simulink model "Shanthan_Heeirthan_EE469S3D_R45 (1)"  (R2023a)
settings: Solver=FixedStepDiscrete  StartTime=0.0  StopTime=120  FixedStep=dt0  RelTol=1e-3  EnableMultiTasking=on
PostLoadFcn:
  | %Set the size for the model
  | set_param(gcs,'Location',[10 10 1270 970])
  | %Set the zoom factor for the model
  | set_param(gcs,'ZoomFactor','100')
InitFcn:
  | tic
  | % Students Add call to their M-file HERE
  | Shanthan_Heeirthan_EE460_Final
  | INIT_S3D_01
StartFcn:
  | tend0=toc;
  | tic;
StopFcn:
  | tend=toc;
  | disp(['Simulation time = ' num2str(tout(end)) ' sec'])
  | disp(['Real time = ' num2str(tend) ' sec'])
  | title('DONE')
  | SCORE=round((max(0,120-tout(end)-tend0))*4+10*(40-FuelBurned)+sum(100*double(PDONE)-100*double(PDONE<.5)));
  | PlotS3D(PlotInput);
  | text(15,22,['S: ' num2str(SCORE)]);
values from neighbouring files (symbols this model uses):
  A = [0 1 0 0 0 0 ... (first row only)    [Shanthan_Heeirthan_EE460_Final (1).m]
  B = [0 0 0 ... (first row only)    [Shanthan_Heeirthan_EE460_Final (1).m]
  bm = [1 1 -1 -1 0 0 0 0; 0 0 0 0 -1 1 1 -1; -1 1 -1 1 3 -3 3 -3]    [Shanthan_Heeirthan_EE460_Final (1).m]
  C = [1 0 0 0 0 0 ... (first row only)    [Shanthan_Heeirthan_EE460_Final (1).m]
  D = [0 0 0 ... (first row only)    [Shanthan_Heeirthan_EE460_Final (1).m]
  Denchptheta = TFchptheta.Den{1}    [Shanthan_Heeirthan_EE460_Final (1).m]
  Denchpxy = TFchpxy.Den{1}    [Shanthan_Heeirthan_EE460_Final (1).m]
  Denclptheta = TFclptheta.Den{1}    [Shanthan_Heeirthan_EE460_Final (1).m]
  Denclpxy = TFclpxy.Den{1}    [Shanthan_Heeirthan_EE460_Final (1).m]
  Denlp = TFlp.Den{1}    [Shanthan_Heeirthan_EE460_Final (1).m]
  Kd = 2.1+0    (= 2.1)    [Shanthan_Heeirthan_EE460_Final (1).m]
  Ki = 0.0001    [Shanthan_Heeirthan_EE460_Final (1).m]
  Kp = 1.1+0.2    (= 1.3)    [Shanthan_Heeirthan_EE460_Final (1).m]
  L = place(A',C',ep)'    [Shanthan_Heeirthan_EE460_Final (1).m]
  Numchptheta = TFchptheta.Num{1}    [Shanthan_Heeirthan_EE460_Final (1).m]
  Numchpxy = TFchpxy.Num{1}    [Shanthan_Heeirthan_EE460_Final (1).m]
  Numclptheta = TFclptheta.Num{1}    [Shanthan_Heeirthan_EE460_Final (1).m]
  Numclpxy = TFclpxy.Num{1}    [Shanthan_Heeirthan_EE460_Final (1).m]
  Numlp = TFlp.Num{1}    [Shanthan_Heeirthan_EE460_Final (1).m]
  Pnewdata = [LVL.P1 LVL.P2 LVL.P3 LVL.P4]    [Shanthan_Heeirthan_EE460_Final (1).m]
  Sconfig = 1    [Shanthan_Heeirthan_EE460_Final (1).m]
  TFP1 = 2    [Shanthan_Heeirthan_EE460_Final (1).m]
  TFP1z = 1    [Shanthan_Heeirthan_EE460_Final (1).m]
  TFP2 = 2    [Shanthan_Heeirthan_EE460_Final (1).m]
  TFP2z = 1    [Shanthan_Heeirthan_EE460_Final (1).m]
  TFP3 = 2    [Shanthan_Heeirthan_EE460_Final (1).m]
  TFP3z = 1    [Shanthan_Heeirthan_EE460_Final (1).m]
  TFP4 = 2    [Shanthan_Heeirthan_EE460_Final (1).m]
  TFP4z = 1    [Shanthan_Heeirthan_EE460_Final (1).m]
  wcf = 2    [Shanthan_Heeirthan_EE460_Final (1).m]
  wcft = 10    [Shanthan_Heeirthan_EE460_Final (1).m]
undefined symbols (not defined in the file or in its folder): d2r, DiscIntNeverNeededParam, dt, dt0, fr, HM_S, HM_U, J, Jbase, JC0, L13, L24, LVL, M, M1, M2, M3, M4, mdti, Pdata, PTvec, r2d, SLIM, SQ, SSF, TOLdata, ULIM
libraries: simulink x85, aerolibanimutils x1, matrix_library x1
(part 4 of 7)

== system Shanthan_Heeirthan_EE469S3D_R45 (1)/S3D_Plant/Sensors/HealthMonitoring/Subsystem2 ==
  In1 : Inport
  Compare To Constant : simulink/Logic and Bit Operations/Compare To Constant  relop=>=  const=HM_S  OutDataTypeStr=boolean
  Constant : Constant  Value=0
  Constant1 : Constant
  Logical Operator : Logic  Operator=OR  AllPortsSameDT=off  OutDataTypeStr=boolean
  Sum : Sum  Inputs=|+-  OutDataTypeStr=int32
  Sum1 : Sum  Inputs=|++
  Switch : Switch  Criteria=u2 > Threshold  Threshold=eps  SaturateOnIntegerOverflow=off  InputSameDT=off
  Unit Delay : UnitDelay  SampleTime=dt0  HasFrameUpgradeWarning=on
  Unit Delay1 : UnitDelay  SampleTime=dt0  HasFrameUpgradeWarning=on
  Unit Delay2 : UnitDelay  SampleTime=dt0  HasFrameUpgradeWarning=on
  Out1 : Outport
  wires:
  Logical Operator/1 -> Unit Delay2/1, Out1/1
  Constant1/1 -> Sum1/1
  Compare To Constant/1 -> Logical Operator/1
  Switch/1 -> Unit Delay1/1, Compare To Constant/1
  In1/1 -> Sum/1, Unit Delay/1
  Unit Delay2/1 -> Logical Operator/2
  Unit Delay/1 -> Sum/2
  Sum/1 -> Switch/2
  Sum1/1 -> Switch/3
  Unit Delay1/1 -> Sum1/2
  Constant/1 -> Switch/1

== system Shanthan_Heeirthan_EE469S3D_R45 (1)/S3D_Plant/Sensors/HealthMonitoring/Subsystem3 ==
  In1 : Inport
  Compare To Constant : simulink/Logic and Bit Operations/Compare To Constant  relop=>=  const=HM_S  OutDataTypeStr=boolean
  Constant : Constant  Value=0
  Constant1 : Constant
  Logical Operator : Logic  Operator=OR  AllPortsSameDT=off  OutDataTypeStr=boolean
  Sum : Sum  Inputs=|+-  OutDataTypeStr=int32
  Sum1 : Sum  Inputs=|++
  Switch : Switch  Criteria=u2 > Threshold  Threshold=eps  SaturateOnIntegerOverflow=off  InputSameDT=off
  Unit Delay : UnitDelay  SampleTime=dt0  HasFrameUpgradeWarning=on
  Unit Delay1 : UnitDelay  SampleTime=dt0  HasFrameUpgradeWarning=on
  Unit Delay2 : UnitDelay  SampleTime=dt0  HasFrameUpgradeWarning=on
  Out1 : Outport
  wires:
  Constant/1 -> Switch/1
  Unit Delay1/1 -> Sum1/2
  Sum1/1 -> Switch/3
  Sum/1 -> Switch/2
  Unit Delay/1 -> Sum/2
  Unit Delay2/1 -> Logical Operator/2
  In1/1 -> Unit Delay/1, Sum/1
  Switch/1 -> Compare To Constant/1, Unit Delay1/1
  Compare To Constant/1 -> Logical Operator/1
  Constant1/1 -> Sum1/1
  Logical Operator/1 -> Out1/1, Unit Delay2/1

== system Shanthan_Heeirthan_EE469S3D_R45 (1)/S3D_Plant/Sensors/HealthMonitoring/Subsystem4 ==
  In1 : Inport
  Compare To Constant : simulink/Logic and Bit Operations/Compare To Constant  relop=>=  const=HM_S  OutDataTypeStr=boolean
  Constant : Constant  Value=0
  Constant1 : Constant
  Logical Operator : Logic  Operator=OR  AllPortsSameDT=off  OutDataTypeStr=boolean
  Sum : Sum  Inputs=|+-  OutDataTypeStr=int32
  Sum1 : Sum  Inputs=|++
  Switch : Switch  Criteria=u2 > Threshold  Threshold=eps  SaturateOnIntegerOverflow=off  InputSameDT=off
  Unit Delay : UnitDelay  SampleTime=dt0  HasFrameUpgradeWarning=on
  Unit Delay1 : UnitDelay  SampleTime=dt0  HasFrameUpgradeWarning=on
  Unit Delay2 : UnitDelay  SampleTime=dt0  HasFrameUpgradeWarning=on
  Out1 : Outport
  wires:
  Logical Operator/1 -> Unit Delay2/1, Out1/1
  Constant1/1 -> Sum1/1
  Compare To Constant/1 -> Logical Operator/1
  Switch/1 -> Unit Delay1/1, Compare To Constant/1
  In1/1 -> Sum/1, Unit Delay/1
  Unit Delay2/1 -> Logical Operator/2
  Unit Delay/1 -> Sum/2
  Sum/1 -> Switch/2
  Sum1/1 -> Switch/3
  Unit Delay1/1 -> Sum1/2
  Constant/1 -> Switch/1

== system Shanthan_Heeirthan_EE469S3D_R45 (1)/S3D_Plant/Sensors/HealthMonitoring/Subsystem5 ==
  In1 : Inport
  Compare To Constant : simulink/Logic and Bit Operations/Compare To Constant  relop=>=  const=HM_S  OutDataTypeStr=boolean
  Constant : Constant  Value=0
  Constant1 : Constant
  Logical Operator : Logic  Operator=OR  AllPortsSameDT=off  OutDataTypeStr=boolean
  Sum : Sum  Inputs=|+-  OutDataTypeStr=int32
  Sum1 : Sum  Inputs=|++
  Switch : Switch  Criteria=u2 > Threshold  Threshold=eps  SaturateOnIntegerOverflow=off  InputSameDT=off
  Unit Delay : UnitDelay  SampleTime=dt0  HasFrameUpgradeWarning=on
  Unit Delay1 : UnitDelay  SampleTime=dt0  HasFrameUpgradeWarning=on
  Unit Delay2 : UnitDelay  SampleTime=dt0  HasFrameUpgradeWarning=on
  Out1 : Outport
  wires:
  Constant/1 -> Switch/1
  Unit Delay1/1 -> Sum1/2
  Sum1/1 -> Switch/3
  Sum/1 -> Switch/2
  Unit Delay/1 -> Sum/2
  Unit Delay2/1 -> Logical Operator/2
  In1/1 -> Unit Delay/1, Sum/1
  Switch/1 -> Compare To Constant/1, Unit Delay1/1
  Compare To Constant/1 -> Logical Operator/1
  Constant1/1 -> Sum1/1
  Logical Operator/1 -> Out1/1, Unit Delay2/1

== system Shanthan_Heeirthan_EE469S3D_R45 (1)/S3D_Plant/Sensors/HealthMonitoring/Subsystem6 ==
  In1 : Inport
  Compare To Constant : simulink/Logic and Bit Operations/Compare To Constant  relop=>=  const=HM_S  OutDataTypeStr=boolean
  Constant : Constant  Value=0
  Constant1 : Constant
  Logical Operator : Logic  Operator=OR  AllPortsSameDT=off  OutDataTypeStr=boolean
  Sum : Sum  Inputs=|+-  OutDataTypeStr=int32
  Sum1 : Sum  Inputs=|++
  Switch : Switch  Criteria=u2 > Threshold  Threshold=eps  SaturateOnIntegerOverflow=off  InputSameDT=off
  Unit Delay : UnitDelay  SampleTime=dt0  HasFrameUpgradeWarning=on
  Unit Delay1 : UnitDelay  SampleTime=dt0  HasFrameUpgradeWarning=on
  Unit Delay2 : UnitDelay  SampleTime=dt0  HasFrameUpgradeWarning=on
  Out1 : Outport
  wires:
  Logical Operator/1 -> Unit Delay2/1, Out1/1
  Constant1/1 -> Sum1/1
  Compare To Constant/1 -> Logical Operator/1
  Switch/1 -> Unit Delay1/1, Compare To Constant/1
  In1/1 -> Sum/1, Unit Delay/1
  Unit Delay2/1 -> Logical Operator/2
  Unit Delay/1 -> Sum/2
  Sum/1 -> Switch/2
  Sum1/1 -> Switch/3
  Unit Delay1/1 -> Sum1/2
  Constant/1 -> Switch/1

== system Shanthan_Heeirthan_EE469S3D_R45 (1)/S3D_Plant/Sensors/HealthMonitoring/Subsystem7 ==
  In1 : Inport
  Compare To Constant : simulink/Logic and Bit Operations/Compare To Constant  relop=>=  const=HM_S  OutDataTypeStr=boolean
  Constant : Constant  Value=0
  Constant1 : Constant
  Logical Operator : Logic  Operator=OR  AllPortsSameDT=off  OutDataTypeStr=boolean
  Sum : Sum  Inputs=|+-  OutDataTypeStr=int32
  Sum1 : Sum  Inputs=|++
  Switch : Switch  Criteria=u2 > Threshold  Threshold=eps  SaturateOnIntegerOverflow=off  InputSameDT=off
  Unit Delay : UnitDelay  SampleTime=dt0  HasFrameUpgradeWarning=on
  Unit Delay1 : UnitDelay  SampleTime=dt0  HasFrameUpgradeWarning=on
  Unit Delay2 : UnitDelay  SampleTime=dt0  HasFrameUpgradeWarning=on
  Out1 : Outport
  wires:
  Constant/1 -> Switch/1
  Unit Delay1/1 -> Sum1/2
  Sum1/1 -> Switch/3
  Sum/1 -> Switch/2
  Unit Delay/1 -> Sum/2
  Unit Delay2/1 -> Logical Operator/2
  In1/1 -> Unit Delay/1, Sum/1
  Switch/1 -> Compare To Constant/1, Unit Delay1/1
  Compare To Constant/1 -> Logical Operator/1
  Constant1/1 -> Sum1/1
  Logical Operator/1 -> Out1/1, Unit Delay2/1

== system Shanthan_Heeirthan_EE469S3D_R45 (1)/S3D_Plant/Sensors/HealthMonitoring/Subsystem8 ==
  In1 : Inport
  Compare To Constant : simulink/Logic and Bit Operations/Compare To Constant  relop=>=  const=HM_S  OutDataTypeStr=boolean
  Constant : Constant  Value=0
  Constant1 : Constant
  Logical Operator : Logic  Operator=OR  AllPortsSameDT=off  OutDataTypeStr=boolean
  Sum : Sum  Inputs=|+-  OutDataTypeStr=int32
  Sum1 : Sum  Inputs=|++
  Switch : Switch  Criteria=u2 > Threshold  Threshold=eps  SaturateOnIntegerOverflow=off  InputSameDT=off
  Unit Delay : UnitDelay  SampleTime=dt0  HasFrameUpgradeWarning=on
  Unit Delay1 : UnitDelay  SampleTime=dt0  HasFrameUpgradeWarning=on
  Unit Delay2 : UnitDelay  SampleTime=dt0  HasFrameUpgradeWarning=on
  Out1 : Outport
  wires:
  Logical Operator/1 -> Unit Delay2/1, Out1/1
  Constant1/1 -> Sum1/1
  Compare To Constant/1 -> Logical Operator/1
  Switch/1 -> Unit Delay1/1, Compare To Constant/1
  In1/1 -> Sum/1, Unit Delay/1
  Unit Delay2/1 -> Logical Operator/2
  Unit Delay/1 -> Sum/2
  Sum/1 -> Switch/2
  Sum1/1 -> Switch/3
  Unit Delay1/1 -> Sum1/2
  Constant/1 -> Switch/1

== system Shanthan_Heeirthan_EE469S3D_R45 (1)/S3D_Plant/ThrusterValues/FailModes/Ufail1 ==
  Uin : Inport
  MP : Inport  Port=2
  Bus Selector1 : BusSelector  OutputSignals=U1cmd,U2cmd,U3cmd,U4cmd,U5cmd,U6cmd,U7cmd,U8cmd,U9cmd,U10cmd  OutputAsBus=on
  Bus Selector2 : BusSelector  OutputSignals=MfuelVector
  Bus to Vector2 : BusToVector
  CURRENT : Subsystem  TreatAsAtomicUnit=on
  Compare To Constant2 : simulink/Logic and Bit Operations/Compare To Constant  relop=>  const=eps  OutDataTypeStr=boolean
  Constant2 : Constant  Value=LVL.Uft(Udx,1)+rand*(LVL.Uft(Udx,2)-LVL.Uft(Udx,1))  SampleTime=dt0
  Constant3 : Constant  Value=LVL.Ufail(Udx)  SampleTime=dt0
  Constant4 : Constant  Value=-1  SampleTime=dt0
  Digital Clock : DigitalClock  SampleTime=dt0
  FailLogic : Subsystem
  If : If  IfExpression=u1 < -0.5  ElseIfExpressions=u1 > 0.5 & u1 < 1.5  SampleTime=dt0
  MAX : Subsystem  TreatAsAtomicUnit=on
  MIN : Subsystem  TreatAsAtomicUnit=on
  Merge : Merge  Inputs=3
  Relational Operator : RelationalOperator  Operator=<  OutDataTypeStr=boolean  InputSameDT=off
  Selector1 : Selector  InputPortWidth=4  IndexOptions=Index vector (dialog)  Indices=[Tank]  OutputSizes=1
  Selector2 : Selector  InputPortWidth=10  IndexOptions=Index vector (dialog)  Indices=[Udx]  OutputSizes=1
  Switch : Switch  Criteria=u2 > Threshold  SaturateOnIntegerOverflow=off  InputSameDT=off
  Switch1 : Switch  Criteria=u2 > Threshold  SaturateOnIntegerOverflow=off  InputSameDT=off
  Unit Delay : UnitDelay  SampleTime=dt0  HasFrameUpgradeWarning=on
  Uout : Outport
  wires:
  Selector2/1 -> Switch/1
  Bus to Vector2/1 -> Selector2/1
  FailLogic/1(NoFail) -> Switch/2
  Compare To Constant2/1 -> Switch1/2, FailLogic/2(FuelRemaining)
  Relational Operator/1 -> FailLogic/1(BeforeFail)
  Constant4/1 -> Switch1/3
  Constant3/1 -> Switch1/1
  Selector1/1 -> Compare To Constant2/1
  Bus Selector2/1 -> Selector1/1  "<MfuelVector>"
  MP/1 -> Bus Selector2/1
  Bus Selector1/1 -> Bus to Vector2/1
  Switch/1 -> Unit Delay/1, Uout/1
  Switch1/1 -> If/1, FailLogic/3(FailMode)
  Uin/1 -> Bus Selector1/1
  Merge/1 -> Switch/3
  MIN/1(Out1) -> Merge/1
  CURRENT/1(Out1) -> Merge/3
  Constant2/1 -> Relational Operator/2
  MAX/1(Out1) -> Merge/2
  Unit Delay/1 -> CURRENT/1(In1)
  If/3 -> CURRENT/Action
  Digital Clock/1 -> Relational Operator/1
  If/2 -> MAX/Action
  If/1 -> MIN/Action

== system Shanthan_Heeirthan_EE469S3D_R45 (1)/S3D_Plant/ThrusterValues/FailModes/Ufail10 ==
  Uin : Inport
  Bus Selector1 : BusSelector  OutputSignals=U1cmd,U2cmd,U3cmd,U4cmd,U5cmd,U6cmd,U7cmd,U8cmd,U9cmd,U10cmd  OutputAsBus=on
  Bus to Vector2 : BusToVector
  CURRENT : Subsystem  TreatAsAtomicUnit=on
  Constant1 : Constant  OutDataTypeStr=boolean  SampleTime=dt0
  Constant2 : Constant  Value=LVL.Uft(Udx,1)+rand*(LVL.Uft(Udx,2)-LVL.Uft(Udx,1))  SampleTime=dt0
  Constant3 : Constant  Value=LVL.Ufail(Udx)  SampleTime=dt0
  Constant4 : Constant  Value=-1  SampleTime=dt0
  Digital Clock : DigitalClock  SampleTime=dt0
  FailLogic : Subsystem
  If : If  IfExpression=u1 < -0.5  ElseIfExpressions=u1 > 0.5 & u1 < 1.5  SampleTime=dt0
  MAX : Subsystem  TreatAsAtomicUnit=on
  MIN : Subsystem  TreatAsAtomicUnit=on
  Merge : Merge  Inputs=3
  Relational Operator : RelationalOperator  Operator=<  OutDataTypeStr=boolean  InputSameDT=off
  Selector2 : Selector  InputPortWidth=10  IndexOptions=Index vector (dialog)  Indices=[Udx]  OutputSizes=1
  Switch : Switch  Criteria=u2 > Threshold  SaturateOnIntegerOverflow=off  InputSameDT=off
  Switch1 : Switch  Criteria=u2 > Threshold  SaturateOnIntegerOverflow=off  InputSameDT=off
  Unit Delay : UnitDelay  SampleTime=dt0  HasFrameUpgradeWarning=on
  Uout : Outport
  wires:
  Selector2/1 -> Switch/1
  Bus to Vector2/1 -> Selector2/1
  Bus Selector1/1 -> Bus to Vector2/1
  FailLogic/1(NoFail) -> Switch/2
  Constant1/1 -> Switch1/2, FailLogic/2(FuelRemaining)
  Relational Operator/1 -> FailLogic/1(BeforeFail)
  Constant4/1 -> Switch1/3
  Constant3/1 -> Switch1/1
  Switch/1 -> Unit Delay/1, Uout/1
  Switch1/1 -> If/1, FailLogic/3(FailMode)
  Uin/1 -> Bus Selector1/1
  Merge/1 -> Switch/3
  MIN/1(Out1) -> Merge/1
  CURRENT/1(Out1) -> Merge/3
  Constant2/1 -> Relational Operator/2
  MAX/1(Out1) -> Merge/2
  Unit Delay/1 -> CURRENT/1(In1)
  If/3 -> CURRENT/Action
  Digital Clock/1 -> Relational Operator/1
  If/2 -> MAX/Action
  If/1 -> MIN/Action

== system Shanthan_Heeirthan_EE469S3D_R45 (1)/S3D_Plant/ThrusterValues/FailModes/Ufail2 ==
  Uin : Inport
  MP : Inport  Port=2
  Bus Selector1 : BusSelector  OutputSignals=U1cmd,U2cmd,U3cmd,U4cmd,U5cmd,U6cmd,U7cmd,U8cmd,U9cmd,U10cmd  OutputAsBus=on
  Bus Selector2 : BusSelector  OutputSignals=MfuelVector
  Bus to Vector2 : BusToVector
  CURRENT : Subsystem  TreatAsAtomicUnit=on
  Compare To Constant2 : simulink/Logic and Bit Operations/Compare To Constant  relop=>  const=eps  OutDataTypeStr=boolean
  Constant2 : Constant  Value=LVL.Uft(Udx,1)+rand*(LVL.Uft(Udx,2)-LVL.Uft(Udx,1))  SampleTime=dt0
  Constant3 : Constant  Value=LVL.Ufail(Udx)  SampleTime=dt0
  Constant4 : Constant  Value=-1  SampleTime=dt0
  Digital Clock : DigitalClock  SampleTime=dt0
  FailLogic : Subsystem
  If : If  IfExpression=u1 < -0.5  ElseIfExpressions=u1 > 0.5 & u1 < 1.5  SampleTime=dt0
  MAX : Subsystem  TreatAsAtomicUnit=on
  MIN : Subsystem  TreatAsAtomicUnit=on
  Merge : Merge  Inputs=3
  Relational Operator : RelationalOperator  Operator=<  OutDataTypeStr=boolean  InputSameDT=off
  Selector1 : Selector  InputPortWidth=4  IndexOptions=Index vector (dialog)  Indices=[Tank]  OutputSizes=1
  Selector2 : Selector  InputPortWidth=10  IndexOptions=Index vector (dialog)  Indices=[Udx]  OutputSizes=1
  Switch : Switch  Criteria=u2 > Threshold  SaturateOnIntegerOverflow=off  InputSameDT=off
  Switch1 : Switch  Criteria=u2 > Threshold  SaturateOnIntegerOverflow=off  InputSameDT=off
  Unit Delay : UnitDelay  SampleTime=dt0  HasFrameUpgradeWarning=on
  Uout : Outport
  wires:
  Selector2/1 -> Switch/1
  Bus to Vector2/1 -> Selector2/1
  Bus Selector1/1 -> Bus to Vector2/1
  FailLogic/1(NoFail) -> Switch/2
  Compare To Constant2/1 -> Switch1/2, FailLogic/2(FuelRemaining)
  Relational Operator/1 -> FailLogic/1(BeforeFail)
  Constant4/1 -> Switch1/3
  Constant3/1 -> Switch1/1
  Selector1/1 -> Compare To Constant2/1
  Bus Selector2/1 -> Selector1/1  "<MfuelVector>"
  MP/1 -> Bus Selector2/1
  Switch/1 -> Unit Delay/1, Uout/1
  Switch1/1 -> If/1, FailLogic/3(FailMode)
  Uin/1 -> Bus Selector1/1
  Merge/1 -> Switch/3
  MIN/1(Out1) -> Merge/1
  CURRENT/1(Out1) -> Merge/3
  Constant2/1 -> Relational Operator/2
  MAX/1(Out1) -> Merge/2
  Unit Delay/1 -> CURRENT/1(In1)
  If/3 -> CURRENT/Action
  Digital Clock/1 -> Relational Operator/1
  If/2 -> MAX/Action
  If/1 -> MIN/Action

== system Shanthan_Heeirthan_EE469S3D_R45 (1)/S3D_Plant/ThrusterValues/FailModes/Ufail3 ==
  Uin : Inport
  MP : Inport  Port=2
  Bus Selector1 : BusSelector  OutputSignals=U1cmd,U2cmd,U3cmd,U4cmd,U5cmd,U6cmd,U7cmd,U8cmd,U9cmd,U10cmd  OutputAsBus=on
  Bus Selector2 : BusSelector  OutputSignals=MfuelVector
  Bus to Vector2 : BusToVector
  CURRENT : Subsystem  TreatAsAtomicUnit=on
  Compare To Constant2 : simulink/Logic and Bit Operations/Compare To Constant  relop=>  const=eps  OutDataTypeStr=boolean
  Constant2 : Constant  Value=LVL.Uft(Udx,1)+rand*(LVL.Uft(Udx,2)-LVL.Uft(Udx,1))  SampleTime=dt0
  Constant3 : Constant  Value=LVL.Ufail(Udx)  SampleTime=dt0
  Constant4 : Constant  Value=-1  SampleTime=dt0
  Digital Clock : DigitalClock  SampleTime=dt0
  FailLogic : Subsystem
  If : If  IfExpression=u1 < -0.5  ElseIfExpressions=u1 > 0.5 & u1 < 1.5  SampleTime=dt0
  MAX : Subsystem  TreatAsAtomicUnit=on
  MIN : Subsystem  TreatAsAtomicUnit=on
  Merge : Merge  Inputs=3
  Relational Operator : RelationalOperator  Operator=<  OutDataTypeStr=boolean  InputSameDT=off
  Selector1 : Selector  InputPortWidth=4  IndexOptions=Index vector (dialog)  Indices=[Tank]  OutputSizes=1
  Selector2 : Selector  InputPortWidth=10  IndexOptions=Index vector (dialog)  Indices=[Udx]  OutputSizes=1
  Switch : Switch  Criteria=u2 > Threshold  SaturateOnIntegerOverflow=off  InputSameDT=off
  Switch1 : Switch  Criteria=u2 > Threshold  SaturateOnIntegerOverflow=off  InputSameDT=off
  Unit Delay : UnitDelay  SampleTime=dt0  HasFrameUpgradeWarning=on
  Uout : Outport
  wires:
  Selector2/1 -> Switch/1
  Bus to Vector2/1 -> Selector2/1
  Bus Selector1/1 -> Bus to Vector2/1
  FailLogic/1(NoFail) -> Switch/2
  Compare To Constant2/1 -> Switch1/2, FailLogic/2(FuelRemaining)
  Relational Operator/1 -> FailLogic/1(BeforeFail)
  Constant4/1 -> Switch1/3
  Constant3/1 -> Switch1/1
  Selector1/1 -> Compare To Constant2/1
  Bus Selector2/1 -> Selector1/1  "<MfuelVector>"
  MP/1 -> Bus Selector2/1
  Switch/1 -> Unit Delay/1, Uout/1
  Switch1/1 -> If/1, FailLogic/3(FailMode)
  Uin/1 -> Bus Selector1/1
  Merge/1 -> Switch/3
  MIN/1(Out1) -> Merge/1
  CURRENT/1(Out1) -> Merge/3
  Constant2/1 -> Relational Operator/2
  MAX/1(Out1) -> Merge/2
  Unit Delay/1 -> CURRENT/1(In1)
  If/3 -> CURRENT/Action
  Digital Clock/1 -> Relational Operator/1
  If/2 -> MAX/Action
  If/1 -> MIN/Action

== system Shanthan_Heeirthan_EE469S3D_R45 (1)/S3D_Plant/ThrusterValues/FailModes/Ufail4 ==
  Uin : Inport
  MP : Inport  Port=2
  Bus Selector1 : BusSelector  OutputSignals=U1cmd,U2cmd,U3cmd,U4cmd,U5cmd,U6cmd,U7cmd,U8cmd,U9cmd,U10cmd  OutputAsBus=on
  Bus Selector2 : BusSelector  OutputSignals=MfuelVector
  Bus to Vector2 : BusToVector
  CURRENT : Subsystem  TreatAsAtomicUnit=on
  Compare To Constant2 : simulink/Logic and Bit Operations/Compare To Constant  relop=>  const=eps  OutDataTypeStr=boolean
  Constant2 : Constant  Value=LVL.Uft(Udx,1)+rand*(LVL.Uft(Udx,2)-LVL.Uft(Udx,1))  SampleTime=dt0
  Constant3 : Constant  Value=LVL.Ufail(Udx)  SampleTime=dt0
  Constant4 : Constant  Value=-1  SampleTime=dt0
  Digital Clock : DigitalClock  SampleTime=dt0
  FailLogic : Subsystem
  If : If  IfExpression=u1 < -0.5  ElseIfExpressions=u1 > 0.5 & u1 < 1.5  SampleTime=dt0
  MAX : Subsystem  TreatAsAtomicUnit=on
  MIN : Subsystem  TreatAsAtomicUnit=on
  Merge : Merge  Inputs=3
  Relational Operator : RelationalOperator  Operator=<  OutDataTypeStr=boolean  InputSameDT=off
  Selector1 : Selector  InputPortWidth=4  IndexOptions=Index vector (dialog)  Indices=[Tank]  OutputSizes=1
  Selector2 : Selector  InputPortWidth=10  IndexOptions=Index vector (dialog)  Indices=[Udx]  OutputSizes=1
  Switch : Switch  Criteria=u2 > Threshold  SaturateOnIntegerOverflow=off  InputSameDT=off
  Switch1 : Switch  Criteria=u2 > Threshold  SaturateOnIntegerOverflow=off  InputSameDT=off
  Unit Delay : UnitDelay  SampleTime=dt0  HasFrameUpgradeWarning=on
  Uout : Outport
  wires:
  Selector2/1 -> Switch/1
  Bus to Vector2/1 -> Selector2/1
  Bus Selector1/1 -> Bus to Vector2/1
  FailLogic/1(NoFail) -> Switch/2
  Compare To Constant2/1 -> Switch1/2, FailLogic/2(FuelRemaining)
  Relational Operator/1 -> FailLogic/1(BeforeFail)
  Constant4/1 -> Switch1/3
  Constant3/1 -> Switch1/1
  Selector1/1 -> Compare To Constant2/1
  Bus Selector2/1 -> Selector1/1  "<MfuelVector>"
  MP/1 -> Bus Selector2/1
  Switch/1 -> Unit Delay/1, Uout/1
  Switch1/1 -> If/1, FailLogic/3(FailMode)
  Uin/1 -> Bus Selector1/1
  Merge/1 -> Switch/3
  MIN/1(Out1) -> Merge/1
  CURRENT/1(Out1) -> Merge/3
  Constant2/1 -> Relational Operator/2
  MAX/1(Out1) -> Merge/2
  Unit Delay/1 -> CURRENT/1(In1)
  If/3 -> CURRENT/Action
  Digital Clock/1 -> Relational Operator/1
  If/2 -> MAX/Action
  If/1 -> MIN/Action

== system Shanthan_Heeirthan_EE469S3D_R45 (1)/S3D_Plant/ThrusterValues/FailModes/Ufail5 ==
  Uin : Inport
  MP : Inport  Port=2
  Bus Selector1 : BusSelector  OutputSignals=U1cmd,U2cmd,U3cmd,U4cmd,U5cmd,U6cmd,U7cmd,U8cmd,U9cmd,U10cmd  OutputAsBus=on
  Bus Selector2 : BusSelector  OutputSignals=MfuelVector
  Bus to Vector2 : BusToVector
  CURRENT : Subsystem  TreatAsAtomicUnit=on
  Compare To Constant2 : simulink/Logic and Bit Operations/Compare To Constant  relop=>  const=eps  OutDataTypeStr=boolean
  Constant2 : Constant  Value=LVL.Uft(Udx,1)+rand*(LVL.Uft(Udx,2)-LVL.Uft(Udx,1))  SampleTime=dt0
  Constant3 : Constant  Value=LVL.Ufail(Udx)  SampleTime=dt0
  Constant4 : Constant  Value=-1  SampleTime=dt0
  Digital Clock : DigitalClock  SampleTime=dt0
  FailLogic : Subsystem
  If : If  IfExpression=u1 < -0.5  ElseIfExpressions=u1 > 0.5 & u1 < 1.5  SampleTime=dt0
  MAX : Subsystem  TreatAsAtomicUnit=on
  MIN : Subsystem  TreatAsAtomicUnit=on
  Merge : Merge  Inputs=3
  Relational Operator : RelationalOperator  Operator=<  OutDataTypeStr=boolean  InputSameDT=off
  Selector1 : Selector  InputPortWidth=4  IndexOptions=Index vector (dialog)  Indices=[Tank]  OutputSizes=1
  Selector2 : Selector  InputPortWidth=10  IndexOptions=Index vector (dialog)  Indices=[Udx]  OutputSizes=1
  Switch : Switch  Criteria=u2 > Threshold  SaturateOnIntegerOverflow=off  InputSameDT=off
  Switch1 : Switch  Criteria=u2 > Threshold  SaturateOnIntegerOverflow=off  InputSameDT=off
  Unit Delay : UnitDelay  SampleTime=dt0  HasFrameUpgradeWarning=on
  Uout : Outport
  wires:
  Selector2/1 -> Switch/1
  Bus to Vector2/1 -> Selector2/1
  Bus Selector1/1 -> Bus to Vector2/1
  FailLogic/1(NoFail) -> Switch/2
  Compare To Constant2/1 -> Switch1/2, FailLogic/2(FuelRemaining)
  Relational Operator/1 -> FailLogic/1(BeforeFail)
  Constant4/1 -> Switch1/3
  Constant3/1 -> Switch1/1
  Selector1/1 -> Compare To Constant2/1
  Bus Selector2/1 -> Selector1/1  "<MfuelVector>"
  MP/1 -> Bus Selector2/1
  Switch/1 -> Unit Delay/1, Uout/1
  Switch1/1 -> If/1, FailLogic/3(FailMode)
  Uin/1 -> Bus Selector1/1
  Merge/1 -> Switch/3
  MIN/1(Out1) -> Merge/1
  CURRENT/1(Out1) -> Merge/3
  Constant2/1 -> Relational Operator/2
  MAX/1(Out1) -> Merge/2
  Unit Delay/1 -> CURRENT/1(In1)
  If/3 -> CURRENT/Action
  Digital Clock/1 -> Relational Operator/1
  If/2 -> MAX/Action
  If/1 -> MIN/Action

== system Shanthan_Heeirthan_EE469S3D_R45 (1)/S3D_Plant/ThrusterValues/FailModes/Ufail6 ==
  Uin : Inport
  MP : Inport  Port=2
  Bus Selector1 : BusSelector  OutputSignals=U1cmd,U2cmd,U3cmd,U4cmd,U5cmd,U6cmd,U7cmd,U8cmd,U9cmd,U10cmd  OutputAsBus=on
  Bus Selector2 : BusSelector  OutputSignals=MfuelVector
  Bus to Vector2 : BusToVector
  CURRENT : Subsystem  TreatAsAtomicUnit=on
  Compare To Constant2 : simulink/Logic and Bit Operations/Compare To Constant  relop=>  const=eps  OutDataTypeStr=boolean
  Constant2 : Constant  Value=LVL.Uft(Udx,1)+rand*(LVL.Uft(Udx,2)-LVL.Uft(Udx,1))  SampleTime=dt0
  Constant3 : Constant  Value=LVL.Ufail(Udx)  SampleTime=dt0
  Constant4 : Constant  Value=-1  SampleTime=dt0
  Digital Clock : DigitalClock  SampleTime=dt0
  FailLogic : Subsystem
  If : If  IfExpression=u1 < -0.5  ElseIfExpressions=u1 > 0.5 & u1 < 1.5  SampleTime=dt0
  MAX : Subsystem  TreatAsAtomicUnit=on
  MIN : Subsystem  TreatAsAtomicUnit=on
  Merge : Merge  Inputs=3
  Relational Operator : RelationalOperator  Operator=<  OutDataTypeStr=boolean  InputSameDT=off
  Selector1 : Selector  InputPortWidth=4  IndexOptions=Index vector (dialog)  Indices=[Tank]  OutputSizes=1
  Selector2 : Selector  InputPortWidth=10  IndexOptions=Index vector (dialog)  Indices=[Udx]  OutputSizes=1
  Switch : Switch  Criteria=u2 > Threshold  SaturateOnIntegerOverflow=off  InputSameDT=off
  Switch1 : Switch  Criteria=u2 > Threshold  SaturateOnIntegerOverflow=off  InputSameDT=off
  Unit Delay : UnitDelay  SampleTime=dt0  HasFrameUpgradeWarning=on
  Uout : Outport
  wires:
  Selector2/1 -> Switch/1
  Bus to Vector2/1 -> Selector2/1
  Bus Selector1/1 -> Bus to Vector2/1
  FailLogic/1(NoFail) -> Switch/2
  Compare To Constant2/1 -> Switch1/2, FailLogic/2(FuelRemaining)
  Relational Operator/1 -> FailLogic/1(BeforeFail)
  Constant4/1 -> Switch1/3
  Constant3/1 -> Switch1/1
  Selector1/1 -> Compare To Constant2/1
  Bus Selector2/1 -> Selector1/1  "<MfuelVector>"
  MP/1 -> Bus Selector2/1
  Switch/1 -> Unit Delay/1, Uout/1
  Switch1/1 -> If/1, FailLogic/3(FailMode)
  Uin/1 -> Bus Selector1/1
  Merge/1 -> Switch/3
  MIN/1(Out1) -> Merge/1
  CURRENT/1(Out1) -> Merge/3
  Constant2/1 -> Relational Operator/2
  MAX/1(Out1) -> Merge/2
  Unit Delay/1 -> CURRENT/1(In1)
  If/3 -> CURRENT/Action
  Digital Clock/1 -> Relational Operator/1
  If/2 -> MAX/Action
  If/1 -> MIN/Action

== system Shanthan_Heeirthan_EE469S3D_R45 (1)/S3D_Plant/ThrusterValues/FailModes/Ufail7 ==
  Uin : Inport
  MP : Inport  Port=2
  Bus Selector1 : BusSelector  OutputSignals=U1cmd,U2cmd,U3cmd,U4cmd,U5cmd,U6cmd,U7cmd,U8cmd,U9cmd,U10cmd  OutputAsBus=on
  Bus Selector2 : BusSelector  OutputSignals=MfuelVector
  Bus to Vector2 : BusToVector
  CURRENT : Subsystem  TreatAsAtomicUnit=on
  Compare To Constant2 : simulink/Logic and Bit Operations/Compare To Constant  relop=>  const=eps  OutDataTypeStr=boolean
  Constant2 : Constant  Value=LVL.Uft(Udx,1)+rand*(LVL.Uft(Udx,2)-LVL.Uft(Udx,1))  SampleTime=dt0
  Constant3 : Constant  Value=LVL.Ufail(Udx)  SampleTime=dt0
  Constant4 : Constant  Value=-1  SampleTime=dt0
  Digital Clock : DigitalClock  SampleTime=dt0
  FailLogic : Subsystem
  If : If  IfExpression=u1 < -0.5  ElseIfExpressions=u1 > 0.5 & u1 < 1.5  SampleTime=dt0
  MAX : Subsystem  TreatAsAtomicUnit=on
  MIN : Subsystem  TreatAsAtomicUnit=on
  Merge : Merge  Inputs=3
  Relational Operator : RelationalOperator  Operator=<  OutDataTypeStr=boolean  InputSameDT=off
  Selector1 : Selector  InputPortWidth=4  IndexOptions=Index vector (dialog)  Indices=[Tank]  OutputSizes=1
  Selector2 : Selector  InputPortWidth=10  IndexOptions=Index vector (dialog)  Indices=[Udx]  OutputSizes=1
  Switch : Switch  Criteria=u2 > Threshold  SaturateOnIntegerOverflow=off  InputSameDT=off
  Switch1 : Switch  Criteria=u2 > Threshold  SaturateOnIntegerOverflow=off  InputSameDT=off
  Unit Delay : UnitDelay  SampleTime=dt0  HasFrameUpgradeWarning=on
  Uout : Outport
  wires:
  Selector2/1 -> Switch/1
  Bus to Vector2/1 -> Selector2/1
  Bus Selector1/1 -> Bus to Vector2/1
  FailLogic/1(NoFail) -> Switch/2
  Compare To Constant2/1 -> Switch1/2, FailLogic/2(FuelRemaining)
  Relational Operator/1 -> FailLogic/1(BeforeFail)
  Constant4/1 -> Switch1/3
  Constant3/1 -> Switch1/1
  Selector1/1 -> Compare To Constant2/1
  Bus Selector2/1 -> Selector1/1  "<MfuelVector>"
  MP/1 -> Bus Selector2/1
  Switch/1 -> Unit Delay/1, Uout/1
  Switch1/1 -> If/1, FailLogic/3(FailMode)
  Uin/1 -> Bus Selector1/1
  Merge/1 -> Switch/3
  MIN/1(Out1) -> Merge/1
  CURRENT/1(Out1) -> Merge/3
  Constant2/1 -> Relational Operator/2
  MAX/1(Out1) -> Merge/2
  Unit Delay/1 -> CURRENT/1(In1)
  If/3 -> CURRENT/Action
  Digital Clock/1 -> Relational Operator/1
  If/2 -> MAX/Action
  If/1 -> MIN/Action

== system Shanthan_Heeirthan_EE469S3D_R45 (1)/S3D_Plant/ThrusterValues/FailModes/Ufail8 ==
  Uin : Inport
  MP : Inport  Port=2
  Bus Selector1 : BusSelector  OutputSignals=U1cmd,U2cmd,U3cmd,U4cmd,U5cmd,U6cmd,U7cmd,U8cmd,U9cmd,U10cmd  OutputAsBus=on
  Bus Selector2 : BusSelector  OutputSignals=MfuelVector
  Bus to Vector2 : BusToVector
  CURRENT : Subsystem  TreatAsAtomicUnit=on
  Compare To Constant2 : simulink/Logic and Bit Operations/Compare To Constant  relop=>  const=eps  OutDataTypeStr=boolean
  Constant2 : Constant  Value=LVL.Uft(Udx,1)+rand*(LVL.Uft(Udx,2)-LVL.Uft(Udx,1))  SampleTime=dt0
  Constant3 : Constant  Value=LVL.Ufail(Udx)  SampleTime=dt0
  Constant4 : Constant  Value=-1  SampleTime=dt0
  Digital Clock : DigitalClock  SampleTime=dt0
  FailLogic : Subsystem
  If : If  IfExpression=u1 < -0.5  ElseIfExpressions=u1 > 0.5 & u1 < 1.5  SampleTime=dt0
  MAX : Subsystem  TreatAsAtomicUnit=on
  MIN : Subsystem  TreatAsAtomicUnit=on
  Merge : Merge  Inputs=3
  Relational Operator : RelationalOperator  Operator=<  OutDataTypeStr=boolean  InputSameDT=off
  Selector1 : Selector  InputPortWidth=4  IndexOptions=Index vector (dialog)  Indices=[Tank]  OutputSizes=1
  Selector2 : Selector  InputPortWidth=10  IndexOptions=Index vector (dialog)  Indices=[Udx]  OutputSizes=1
  Switch : Switch  Criteria=u2 > Threshold  SaturateOnIntegerOverflow=off  InputSameDT=off
  Switch1 : Switch  Criteria=u2 > Threshold  SaturateOnIntegerOverflow=off  InputSameDT=off
  Unit Delay : UnitDelay  SampleTime=dt0  HasFrameUpgradeWarning=on
  Uout : Outport
  wires:
  Selector2/1 -> Switch/1
  Bus to Vector2/1 -> Selector2/1
  Bus Selector1/1 -> Bus to Vector2/1
  FailLogic/1(NoFail) -> Switch/2
  Compare To Constant2/1 -> Switch1/2, FailLogic/2(FuelRemaining)
  Relational Operator/1 -> FailLogic/1(BeforeFail)
  Constant4/1 -> Switch1/3
  Constant3/1 -> Switch1/1
  Selector1/1 -> Compare To Constant2/1
  Bus Selector2/1 -> Selector1/1  "<MfuelVector>"
  MP/1 -> Bus Selector2/1
  Switch/1 -> Unit Delay/1, Uout/1
  Switch1/1 -> If/1, FailLogic/3(FailMode)
  Uin/1 -> Bus Selector1/1
  Merge/1 -> Switch/3
  MIN/1(Out1) -> Merge/1
  CURRENT/1(Out1) -> Merge/3
  Constant2/1 -> Relational Operator/2
  MAX/1(Out1) -> Merge/2
  Unit Delay/1 -> CURRENT/1(In1)
  If/3 -> CURRENT/Action
  Digital Clock/1 -> Relational Operator/1
  If/2 -> MAX/Action
  If/1 -> MIN/Action

== system Shanthan_Heeirthan_EE469S3D_R45 (1)/S3D_Plant/ThrusterValues/FailModes/Ufail9 ==
  Uin : Inport
  Bus Selector1 : BusSelector  OutputSignals=U1cmd,U2cmd,U3cmd,U4cmd,U5cmd,U6cmd,U7cmd,U8cmd,U9cmd,U10cmd  OutputAsBus=on
  Bus to Vector2 : BusToVector
  CURRENT : Subsystem  TreatAsAtomicUnit=on
  Constant2 : Constant  Value=LVL.Uft(Udx,1)+rand*(LVL.Uft(Udx,2)-LVL.Uft(Udx,1))  SampleTime=dt0
  Constant3 : Constant  Value=LVL.Ufail(Udx)  SampleTime=dt0
  Constant4 : Constant  Value=-1  SampleTime=dt0
  Constant5 : Constant  OutDataTypeStr=boolean  SampleTime=dt0
  Digital Clock : DigitalClock  SampleTime=dt0
  FailLogic : Subsystem
  If : If  IfExpression=u1 < -0.5  ElseIfExpressions=u1 > 0.5 & u1 < 1.5  SampleTime=dt0
  MAX : Subsystem  TreatAsAtomicUnit=on
  MIN : Subsystem  TreatAsAtomicUnit=on
  Merge : Merge  Inputs=3
  Relational Operator : RelationalOperator  Operator=<  OutDataTypeStr=boolean  InputSameDT=off
  Selector2 : Selector  InputPortWidth=10  IndexOptions=Index vector (dialog)  Indices=[Udx]  OutputSizes=1
  Switch : Switch  Criteria=u2 > Threshold  SaturateOnIntegerOverflow=off  InputSameDT=off
  Switch1 : Switch  Criteria=u2 > Threshold  SaturateOnIntegerOverflow=off  InputSameDT=off
  Unit Delay : UnitDelay  SampleTime=dt0  HasFrameUpgradeWarning=on
  Uout : Outport
  wires:
  Constant5/1 -> Switch1/2, FailLogic/2(FuelRemaining)
  Selector2/1 -> Switch/1
  Bus to Vector2/1 -> Selector2/1
  Bus Selector1/1 -> Bus to Vector2/1
  FailLogic/1(NoFail) -> Switch/2
  Relational Operator/1 -> FailLogic/1(BeforeFail)
  Constant4/1 -> Switch1/3
  Constant3/1 -> Switch1/1
  Switch/1 -> Unit Delay/1, Uout/1
  Switch1/1 -> If/1, FailLogic/3(FailMode)
  Uin/1 -> Bus Selector1/1
  Merge/1 -> Switch/3
  MIN/1(Out1) -> Merge/1
  CURRENT/1(Out1) -> Merge/3
  Constant2/1 -> Relational Operator/2
  MAX/1(Out1) -> Merge/2
  Unit Delay/1 -> CURRENT/1(In1)
  If/3 -> CURRENT/Action
  Digital Clock/1 -> Relational Operator/1
  If/2 -> MAX/Action
  If/1 -> MIN/Action

== system Shanthan_Heeirthan_EE469S3D_R45 (1)/S3D_Plant/ThrusterValues/HealthMonitoring/DetectFailures ==
  Uvalues : Inport
  UCMD : Inport  Port=2
  Bus Creator : BusCreator  Inputs=2
  Bus Creator1 : BusCreator  Inputs=10
  Bus Selector : BusSelector  OutputSignals=Ucmd.U1cmd,U.U1
  Bus Selector1 : BusSelector  OutputSignals=Ucmd.U2cmd,U.U2
  Bus Selector2 : BusSelector  OutputSignals=Ucmd.U3cmd,U.U3
  Bus Selector3 : BusSelector  OutputSignals=Ucmd.U4cmd,U.U4
  Bus Selector4 : BusSelector  OutputSignals=Ucmd.U5cmd,U.U5
  Bus Selector5 : BusSelector  OutputSignals=Ucmd.U6cmd,U.U6
  Bus Selector6 : BusSelector  OutputSignals=Ucmd.U7cmd,U.U7
  Bus Selector7 : BusSelector  OutputSignals=Ucmd.U8cmd,U.U8
  Bus Selector8 : BusSelector  OutputSignals=Ucmd.U9cmd,U.U9
  Bus Selector9 : BusSelector  OutputSignals=Ucmd.U10cmd,U.U10
  Subsystem : Subsystem
  Subsystem1 : Subsystem
  Subsystem2 : Subsystem
  Subsystem3 : Subsystem
  Subsystem4 : Subsystem
  Subsystem5 : Subsystem
  Subsystem6 : Subsystem
  Subsystem7 : Subsystem
  Subsystem8 : Subsystem
  Subsystem9 : Subsystem
  Out2 : Outport
  wires:
  Subsystem7/1(Out1) -> Bus Creator1/8  "U8fail"
  Bus Creator/1 -> Bus Selector/1, Bus Selector1/1, Bus Selector2/1, Bus Selector3/1, Bus Selector4/1, Bus Selector5/1, Bus Selector6/1, Bus Selector7/1, Bus Selector8/1, Bus Selector9/1
  Subsystem3/1(Out1) -> Bus Creator1/4  "U4fail"
  Subsystem9/1(Out1) -> Bus Creator1/10  "U10fail"
  Subsystem8/1(Out1) -> Bus Creator1/9  "U9fail"
  Subsystem1/1(Out1) -> Bus Creator1/2  "U2fail"
  Bus Selector9/2 -> Subsystem9/2(U)  "<U10>"
  Bus Selector1/1 -> Subsystem1/1(UCMD)  "<U2cmd>"
  Bus Selector8/1 -> Subsystem8/1(UCMD)  "<U9cmd>"
  Bus Selector1/2 -> Subsystem1/2(U)  "<U2>"
  Uvalues/1 -> Bus Creator/2
  Bus Selector6/2 -> Subsystem6/2(U)  "<U7>"
  Subsystem4/1(Out1) -> Bus Creator1/5  "U5fail"
  Bus Selector9/1 -> Subsystem9/1(UCMD)  "<U10cmd>"
  Bus Selector6/1 -> Subsystem6/1(UCMD)  "<U7cmd>"
  Subsystem2/1(Out1) -> Bus Creator1/3  "U3fail"
  Bus Selector3/1 -> Subsystem3/1(UCMD)  "<U4cmd>"
  Bus Selector5/2 -> Subsystem5/2(U)  "<U6>"
  Bus Selector7/1 -> Subsystem7/1(UCMD)  "<U8cmd>"
  Bus Selector8/2 -> Subsystem8/2(U)  "<U9>"
  Bus Selector4/1 -> Subsystem4/1(UCMD)  "<U5cmd>"
  Bus Creator1/1 -> Out2/1  "Ufail"
  Bus Selector5/1 -> Subsystem5/1(UCMD)  "<U6cmd>"
  Bus Selector2/2 -> Subsystem2/2(U)  "<U3>"
  Bus Selector4/2 -> Subsystem4/2(U)  "<U5>"
  Bus Selector3/2 -> Subsystem3/2(U)  "<U4>"
  Subsystem5/1(Out1) -> Bus Creator1/6  "U6fail"
  Bus Selector2/1 -> Subsystem2/1(UCMD)  "<U3cmd>"
  Bus Selector/1 -> Subsystem/1(UCMD)  "<U1cmd>"
  Bus Selector/2 -> Subsystem/2(U)  "<U1>"
  Subsystem6/1(Out1) -> Bus Creator1/7  "U7fail"
  Bus Selector7/2 -> Subsystem7/2(U)  "<U8>"
  Subsystem/1(Out1) -> Bus Creator1/1  "U1fail"
  UCMD/1 -> Bus Creator/1

== system Shanthan_Heeirthan_EE469S3D_R45 (1)/control_law/CMD/CMDprocess/CommandTypes ==
  Pdata : Inport
  Point : Inport  Port=2
  Sensed : Inport  Port=3
  Bus Creator : BusCreator  Inputs=3
  Bus Creator1 : BusCreator  Inputs=3
  Bus Creator2 : BusCreator  Inputs=3
  Demux : Demux  Outputs=3
  Demux1 : Demux  Outputs=3
  Enabled Subsystem : Subsystem  TreatAsAtomicUnit=on
  If : If  IfExpression=u1 < 1.5  ElseIfExpressions=u1<2.5, u1<3.5
  Merge1 : Merge  Inputs=4
  Ramp1 : Subsystem  TreatAsAtomicUnit=on
  Ramp2 : Subsystem  TreatAsAtomicUnit=on
  Ramp3 : Subsystem  TreatAsAtomicUnit=on
  Ramp4 : Subsystem  TreatAsAtomicUnit=on
  Relational Operator : RelationalOperator  Operator=~=  OutDataTypeStr=boolean  RndMeth=Simplest  InputSameDT=off
  Unit Delay : UnitDelay  SampleTime=dt  HasFrameUpgradeWarning=on
  Unit Delay1 : UnitDelay  SampleTime=dt  HasFrameUpgradeWarning=on
  CMDS : Outport
  wires:
  If/2 -> Ramp4/Action
  Pdata/1 -> Demux1/1, Unit Delay1/1
  If/1 -> Ramp1/Action
  If/3 -> Ramp2/Action
  Ramp2/1(RMP_CMDS) -> Merge1/3
  If/4 -> Ramp3/Action
  Merge1/1 -> Demux/1
  Demux/1 -> Bus Creator/1  "X_CMD"
  Demux/2 -> Bus Creator/2  "Y_CMD"
  Demux/3 -> Bus Creator/3  "theta_CMD"
  Bus Creator/1 -> CMDS/1  "CMDS"
  Point/1 -> If/1, Relational Operator/1, Unit Delay/1
  Unit Delay/1 -> Relational Operator/2
  Relational Operator/1 -> Enabled Subsystem/Enable
  Unit Delay1/1 -> Enabled Subsystem/1(Pdata)  "Pdata"
  Enabled Subsystem/1(ICs) -> Bus Creator1/1  "ICs"
  Bus Creator1/1 -> Ramp2/1(ICCMDs), Ramp4/1(ICCMDs), Ramp1/1(ICCMDs), Ramp3/1(ICCMDs)  "ICCMDS"
  Demux1/1 -> Bus Creator2/1  "XdesCMD"
  Demux1/2 -> Bus Creator2/2  "YdesCMD"
  Demux1/3 -> Bus Creator2/3  "ZdesCMD"
  Bus Creator2/1 -> Bus Creator1/2  "CMDS"
  Sensed/1 -> Bus Creator1/3
  Ramp1/1(RMP_CMDS) -> Merge1/1
  Ramp4/1(RMP_CMDS) -> Merge1/2
  Ramp3/1(RMP_CMDS) -> Merge1/4

== system Shanthan_Heeirthan_EE469S3D_R45 (1)/control_law/InputDataConditioning/SensorConditioning/JustX ==
  Xsens : Inport
  Bus Selector : BusSelector  OutputSignals=Sensor1,S1fail,Sensor2,S2fail,Sensor3
  Data Type Conversion : DataTypeConversion  OutDataTypeStr=double  SaturateOnIntegerOverflow=off  RndMeth=Floor
  Data Type Conversion1 : DataTypeConversion  OutDataTypeStr=double  SaturateOnIntegerOverflow=off  RndMeth=Floor
  Data Type Conversion2 : DataTypeConversion  OutDataTypeStr=double  SaturateOnIntegerOverflow=off  RndMeth=Floor
  Discrete Transfer Fcn{1..5} (5 alike) : DiscreteTransferFcn  Numerator=Numlp  Denominator=Denlp  SampleTime=dt
  Discrete-Time Integrator : DiscreteIntegrator  SampleTime=-1  ICPrevOutput=DiscIntNeverNeededParam  ICPrevScaledInput=DiscIntNeverNeededParam
  Discrete-Time Integrator1 : DiscreteIntegrator  SampleTime=-1  ICPrevOutput=DiscIntNeverNeededParam  ICPrevScaledInput=DiscIntNeverNeededParam
  Gain : Gain  Gain=0.005
  Gain1 : Gain  Gain=0.01
  Gain2 : Gain  Gain=0.004
  NOT : Logic  Operator=NOT  IconShape=distinctive  AllPortsSameDT=off  OutDataTypeStr=boolean
  NOT1 : Logic  Operator=NOT  IconShape=distinctive  AllPortsSameDT=off  OutDataTypeStr=boolean
  Switch : Switch  Criteria=u2 ~= 0  SaturateOnIntegerOverflow=off  InputSameDT=off
  Switch1 : Switch  Criteria=u2 ~= 0  SaturateOnIntegerOverflow=off  InputSameDT=off
  Unit Delay : UnitDelay  InitialCondition=26  SampleTime=dt  HasFrameUpgradeWarning=on
  Unit Delay1 : UnitDelay  InitialCondition=26  SampleTime=dt  HasFrameUpgradeWarning=on
  xpos : Outport
  xvel : Outport  Port=2
  xacc : Outport  Port=3
  wires:
  Xsens/1 -> Bus Selector/1
  Bus Selector/1 -> Data Type Conversion/1  "<Sensor1>"
  Bus Selector/2 -> NOT/1  "<S1fail>"
  Bus Selector/3 -> Data Type Conversion2/1  "<Sensor2>"
  Discrete-Time Integrator/1 -> Discrete Transfer Fcn2/1
  Switch/1 -> xpos/1  "X1_m"
  Bus Selector/4 -> NOT1/1  "<S2fail>"
  NOT/1 -> Switch/2
  NOT1/1 -> Switch1/2
  Discrete-Time Integrator1/1 -> Discrete Transfer Fcn4/1
  Bus Selector/5 -> Data Type Conversion1/1  "<Sensor3>"
  Switch1/1 -> xvel/1  "X_mps"
  Data Type Conversion/1 -> Gain/1
  Gain/1 -> Discrete Transfer Fcn1/1
  Data Type Conversion2/1 -> Gain1/1
  Gain1/1 -> Discrete Transfer Fcn3/1, Unit Delay/1  "X_mps"
  Data Type Conversion1/1 -> Gain2/1
  Gain2/1 -> Discrete Transfer Fcn5/1, Unit Delay1/1  "X_mps2"
  Unit Delay/1 -> Discrete-Time Integrator/1
  Unit Delay1/1 -> Discrete-Time Integrator1/1
  Discrete Transfer Fcn2/1 -> Switch/3
  Discrete Transfer Fcn1/1 -> Switch/1
  Discrete Transfer Fcn3/1 -> Switch1/1
  Discrete Transfer Fcn4/1 -> Switch1/3  "X_mps2"
  Discrete Transfer Fcn5/1 -> xacc/1  "X_mps2"

== system Shanthan_Heeirthan_EE469S3D_R45 (1)/control_law/InputDataConditioning/SensorConditioning/JustY ==
  Ysens : Inport
  Bus Selector : BusSelector  OutputSignals=Sensor4,S4fail,Sensor5,S5fail,Sensor6
  Data Type Conversion : DataTypeConversion  OutDataTypeStr=double  SaturateOnIntegerOverflow=off  RndMeth=Floor
  Data Type Conversion1 : DataTypeConversion  OutDataTypeStr=double  SaturateOnIntegerOverflow=off  RndMeth=Floor
  Data Type Conversion2 : DataTypeConversion  OutDataTypeStr=double  SaturateOnIntegerOverflow=off  RndMeth=Floor
  Discrete Transfer Fcn{1..5} (5 alike) : DiscreteTransferFcn  Numerator=Numlp  Denominator=Denlp  SampleTime=dt
  Discrete-Time Integrator : DiscreteIntegrator  SampleTime=-1  ICPrevOutput=DiscIntNeverNeededParam  ICPrevScaledInput=DiscIntNeverNeededParam
  Discrete-Time Integrator1 : DiscreteIntegrator  SampleTime=-1  ICPrevOutput=DiscIntNeverNeededParam  ICPrevScaledInput=DiscIntNeverNeededParam
  Gain : Gain  Gain=0.005
  Gain1 : Gain  Gain=0.01
  Gain2 : Gain  Gain=0.004
  NOT : Logic  Operator=NOT  IconShape=distinctive  AllPortsSameDT=off  OutDataTypeStr=boolean
  NOT1 : Logic  Operator=NOT  IconShape=distinctive  AllPortsSameDT=off  OutDataTypeStr=boolean
  Switch : Switch  Criteria=u2 ~= 0  SaturateOnIntegerOverflow=off  InputSameDT=off
  Switch1 : Switch  Criteria=u2 ~= 0  SaturateOnIntegerOverflow=off  InputSameDT=off
  Unit Delay1 : UnitDelay  InitialCondition=26  SampleTime=dt  HasFrameUpgradeWarning=on
  Unit Delay2 : UnitDelay  InitialCondition=26  SampleTime=dt  HasFrameUpgradeWarning=on
  ypos : Outport
  yvel : Outport  Port=2
  yacc : Outport  Port=3
  wires:
  Gain2/1 -> Discrete Transfer Fcn4/1, Unit Delay1/1
  Bus Selector/2 -> NOT/1  "<S4fail>"
  Switch1/1 -> yvel/1  "Y_mps"
  Switch/1 -> ypos/1  "Y_m"
  Data Type Conversion2/1 -> Gain1/1
  Discrete-Time Integrator/1 -> Discrete Transfer Fcn2/1
  Data Type Conversion1/1 -> Gain2/1
  Data Type Conversion/1 -> Gain/1
  Bus Selector/5 -> Data Type Conversion1/1  "<Sensor6>"
  Gain/1 -> Discrete Transfer Fcn1/1
  NOT/1 -> Switch/2
  NOT1/1 -> Switch1/2
  Gain1/1 -> Discrete Transfer Fcn3/1, Unit Delay2/1
  Bus Selector/4 -> NOT1/1  "<S5fail>"
  Discrete-Time Integrator1/1 -> Discrete Transfer Fcn5/1
  Bus Selector/3 -> Data Type Conversion2/1  "<Sensor5>"
  Ysens/1 -> Bus Selector/1
  Bus Selector/1 -> Data Type Conversion/1  "<Sensor4>"
  Unit Delay1/1 -> Discrete-Time Integrator1/1
  Unit Delay2/1 -> Discrete-Time Integrator/1
  Discrete Transfer Fcn2/1 -> Switch/3
  Discrete Transfer Fcn1/1 -> Switch/1
  Discrete Transfer Fcn3/1 -> Switch1/1
  Discrete Transfer Fcn4/1 -> yacc/1  "Y_mps2"
  Discrete Transfer Fcn5/1 -> Switch1/3

== system Shanthan_Heeirthan_EE469S3D_R45 (1)/control_law/InputDataConditioning/SensorConditioning/JustZ ==
  Zsens : Inport
  Bus Selector : BusSelector  OutputSignals=Sensor7,S7fail,Sensor8,S8fail,Sensor9
  Data Type Conversion : DataTypeConversion  OutDataTypeStr=double  SaturateOnIntegerOverflow=off  RndMeth=Floor
  Data Type Conversion1 : DataTypeConversion  OutDataTypeStr=double  SaturateOnIntegerOverflow=off  RndMeth=Floor
  Data Type Conversion2 : DataTypeConversion  OutDataTypeStr=double  SaturateOnIntegerOverflow=off  RndMeth=Floor
  Discrete Transfer Fcn{1..5} (5 alike) : DiscreteTransferFcn  Numerator=Numlp  Denominator=Denlp  SampleTime=dt
  Discrete-Time Integrator : DiscreteIntegrator  SampleTime=-1  ICPrevOutput=DiscIntNeverNeededParam  ICPrevScaledInput=DiscIntNeverNeededParam
  Discrete-Time Integrator1 : DiscreteIntegrator  SampleTime=-1  ICPrevOutput=DiscIntNeverNeededParam  ICPrevScaledInput=DiscIntNeverNeededParam
  Gain : Gain  Gain=0.02
  Gain1 : Gain  Gain=0.01
  Gain2 : Gain  Gain=0.004
  NOT : Logic  Operator=NOT  IconShape=distinctive  AllPortsSameDT=off  OutDataTypeStr=boolean
  NOT1 : Logic  Operator=NOT  IconShape=distinctive  AllPortsSameDT=off  OutDataTypeStr=boolean
  Switch : Switch  Criteria=u2 ~= 0  SaturateOnIntegerOverflow=off  InputSameDT=off
  Switch1 : Switch  Criteria=u2 ~= 0  SaturateOnIntegerOverflow=off  InputSameDT=off
  Unit Delay1 : UnitDelay  InitialCondition=26  SampleTime=dt  HasFrameUpgradeWarning=on
  Unit Delay2 : UnitDelay  InitialCondition=26  SampleTime=dt  HasFrameUpgradeWarning=on
  thetapos : Outport
  thetavel : Outport  Port=2
  thetaacc : Outport  Port=3
  wires:
  Zsens/1 -> Bus Selector/1
  Switch1/1 -> thetavel/1  "theta_degps"
  Data Type Conversion2/1 -> Gain1/1
  Discrete-Time Integrator/1 -> Discrete Transfer Fcn2/1
  Gain/1 -> Discrete Transfer Fcn4/1
  Gain2/1 -> Discrete Transfer Fcn3/1, Unit Delay2/1  "theta_degps2"
  Bus Selector/2 -> NOT/1  "<S7fail>"
  NOT1/1 -> Switch1/2
  NOT/1 -> Switch/2
  Gain1/1 -> Discrete Transfer Fcn5/1, Unit Delay1/1
  Bus Selector/5 -> Data Type Conversion1/1  "<Sensor9>"
  Data Type Conversion/1 -> Gain/1
  Bus Selector/3 -> Data Type Conversion2/1  "<Sensor8>"
  Bus Selector/1 -> Data Type Conversion/1  "<Sensor7>"
  Discrete-Time Integrator1/1 -> Discrete Transfer Fcn1/1
  Bus Selector/4 -> NOT1/1  "<S8fail>"
  Switch/1 -> thetapos/1  "theta_deg"
  Data Type Conversion1/1 -> Gain2/1
  Unit Delay1/1 -> Discrete-Time Integrator/1
  Unit Delay2/1 -> Discrete-Time Integrator1/1
  Discrete Transfer Fcn2/1 -> Switch/3
  Discrete Transfer Fcn1/1 -> Switch1/3
  Discrete Transfer Fcn3/1 -> thetaacc/1  "theta_degps2"
  Discrete Transfer Fcn4/1 -> Switch/1
  Discrete Transfer Fcn5/1 -> Switch1/1

== system Shanthan_Heeirthan_EE469S3D_R45 (1)/control_law/thrustercmd/GenInverse/WeightedMatrix ==
  Ufail : Inport
  Bus to Vector : BusToVector
  Constant : Constant  Value=eye(8)
  Create Diagonal Matrix : matrix_library/Create Diagonal Matrix
      settings: LibrarySourceBlock=|
      | simulink/Matrix
      | Operations/Create Diagonal
      | Matrix
  Data Type Conversion : DataTypeConversion  OutDataTypeStr=double  SaturateOnIntegerOverflow=off  RndMeth=Floor
  Gain : Gain  Gain=1000
  Sum : Sum  Inputs=|++
  Weight : Outport
  wires:
  Constant/1 -> Sum/2
  Sum/1 -> Weight/1  "Weight"
  Ufail/1 -> Bus to Vector/1
  Bus to Vector/1 -> Data Type Conversion/1
  Data Type Conversion/1 -> Create Diagonal Matrix/1
  Create Diagonal Matrix/1 -> Gain/1
  Gain/1 -> Sum/1

== system Shanthan_Heeirthan_EE469S3D_R45 (1)/S3D_Plant/Sensors/CASE1/THTaccel/CURRENT ==
  In1 : Inport
  Action Port : ActionPort  ActionPortLabel=else
  Out1 : Outport
  wires:
  In1/1 -> Out1/1

== system Shanthan_Heeirthan_EE469S3D_R45 (1)/S3D_Plant/Sensors/CASE1/THTaccel/MAX ==
  Action Port : ActionPort  ActionPortLabel=elseif(u1 > 0.5 & u1 < 1.5)
  Constant : Constant  Value=SLIM(9,2)  SampleTime=dt0
  Out1 : Outport
  wires:
  Constant/1 -> Out1/1

== system Shanthan_Heeirthan_EE469S3D_R45 (1)/S3D_Plant/Sensors/CASE1/THTaccel/MIN ==
  Action Port : ActionPort  ActionPortLabel=if(u1 < -0.5)
  Constant : Constant  Value=SLIM(9,1)  SampleTime=dt0
  Out1 : Outport
  wires:
  Constant/1 -> Out1/1

== system Shanthan_Heeirthan_EE469S3D_R45 (1)/S3D_Plant/Sensors/CASE1/THTpos1/CURRENT ==
  In1 : Inport
  Action Port : ActionPort  ActionPortLabel=else
  Out1 : Outport
  wires:
  In1/1 -> Out1/1

== system Shanthan_Heeirthan_EE469S3D_R45 (1)/S3D_Plant/Sensors/CASE1/THTpos1/MAX ==
  Action Port : ActionPort  ActionPortLabel=elseif(u1 > 0.5 & u1 < 1.5)
  Constant : Constant  Value=SLIM(7,2)  SampleTime=dt0
  Out1 : Outport
  wires:
  Constant/1 -> Out1/1

== system Shanthan_Heeirthan_EE469S3D_R45 (1)/S3D_Plant/Sensors/CASE1/THTpos1/MIN ==
  Action Port : ActionPort  ActionPortLabel=if(u1 < -0.5)
  Constant : Constant  Value=SLIM(7,1)  SampleTime=dt0
  Out1 : Outport
  wires:
  Constant/1 -> Out1/1

== system Shanthan_Heeirthan_EE469S3D_R45 (1)/S3D_Plant/Sensors/CASE1/THTvel/CURRENT ==
  In1 : Inport
  Action Port : ActionPort  ActionPortLabel=else
  Out1 : Outport
  wires:
  In1/1 -> Out1/1

== system Shanthan_Heeirthan_EE469S3D_R45 (1)/S3D_Plant/Sensors/CASE1/THTvel/MAX ==
  Action Port : ActionPort  ActionPortLabel=elseif(u1 > 0.5 & u1 < 1.5)
  Constant : Constant  Value=SLIM(8,2)  SampleTime=dt0
  Out1 : Outport
  wires:
  Constant/1 -> Out1/1

== system Shanthan_Heeirthan_EE469S3D_R45 (1)/S3D_Plant/Sensors/CASE1/THTvel/MIN ==
  Action Port : ActionPort  ActionPortLabel=if(u1 < -0.5)
  Constant : Constant  Value=SLIM(8,1)  SampleTime=dt0
  Out1 : Outport
  wires:
  Constant/1 -> Out1/1
